simulink model "rl_with_free"  (R2021a)
settings: Solver=ode3  StartTime=0.0  StopTime=no_of_cycles/freq  MaxStep=1e-4  RelTol=1e-3
values from neighbouring files (symbols this model uses):
  firing_angle = c    [control.m]
  freq = a    [control.m]    (also in uncontrolled.m)
  peak_amp = d    [control.m]    (also in uncontrolled.m)
libraries: spsThyristorLib x4, spsACVoltageSourceLib x1, spsCurrentMeasurementLib x1, spsDiodeLib x1, spsSeriesRLCBranchLib x1, spsVoltageMeasurementLib x1, spspowerguiLib x1
settings Model: Creator=Souhardya  LastModifiedBy=sayan
settings SolverCC: AlgebraicLoopSolver=TrustRegion
settings DataIOCC: ReturnWorkspaceOutputs=off
settings DebuggingCC: SFMachineParentedDataDiag=warning  ArithmeticOperatorsInVariantConditions=warning
settings SFSimCC: SimUseLocalCustomCode=off  CustomCodeUndefinedFunction=UseInterfaceOnly
settings RTWCC: RTWUseLocalCustomCode=off
settings CodeAppCC: StateflowObjectComments=on
settings SimscapeCC: SimscapeNormalizeSystem=off

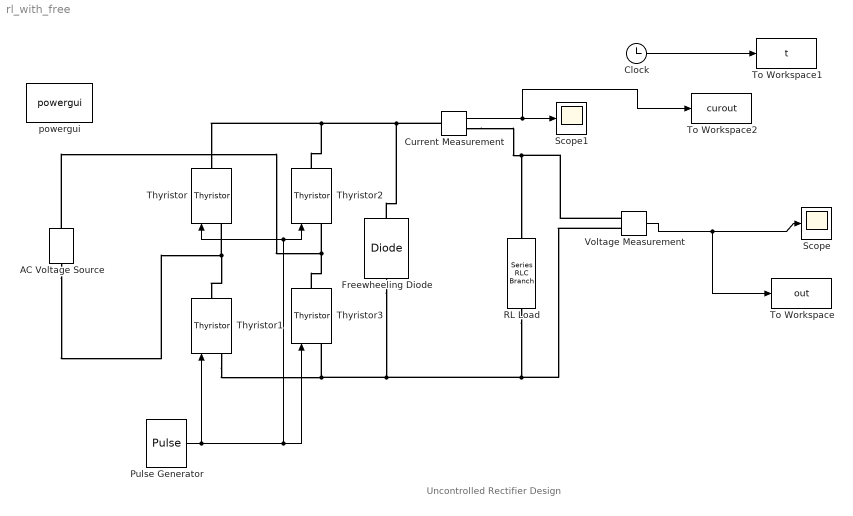
== system rl_with_free ==
  note: Uncontrolled Rectifier Design
  AC Voltage Source : spsACVoltageSourceLib/AC Voltage Source  Amplitude=peak_amp  Phase=0  Frequency=freq  SampleTime=0  Measurements=None  BusType=swing  Pref=10e3  Qref=0  Qmin=-inf  Qmax=+inf
  Clock : Clock
  Current Measurement : spsCurrentMeasurementLib/Current Measurement  PhasorSimulation=off  OutputType=Complex  PSBequivalent=0
  Freewheeling Diode : spsDiodeLib/Diode  Ron=0.001  Lon=0  Vf=0.8  IC=0  UseSnubber=0  Rs=500  Cs=250e-9  Measurements=off
  Pulse Generator : DiscretePulseGenerator  PulseType=Time based  Period=1/(2*freq)  PulseWidth=5  PhaseDelay=((1/freq)/360)*mod(firing_angle,360)
  RL Load : spsSeriesRLCBranchLib/Series RLC Branch  LConnTagsString=__new0  RConnTagsString=__new0  BranchType=RL  Resistance=1  Inductance=5e-2  SetiL0=off  InitialCurrent=0  Capacitance=1e-6  Setx0=off  InitialVoltage=0  Measurements=None
  Scope : Scope
  Scope1 : Scope
  Thyristor{,1..3} (4 alike) : spsThyristorLib/Thyristor  Ron=0.001  Lon=0  Vf=0.8  IC=0  Rs=500  Cs=250e-9  Measurements=off
  To Workspace : ToWorkspace  VariableName=out  SampleTime=-1
  To Workspace1 : ToWorkspace  VariableName=t  SampleTime=-1
  To Workspace2 : ToWorkspace  VariableName=curout  SampleTime=-1
  Voltage Measurement : spsVoltageMeasurementLib/Voltage Measurement  PhasorSimulation=off  OutputType=Complex  PSBequivalent=0
  powergui : spspowerguiLib/powergui  Priority=1  SimulationMode=Continuous  SampleTime=50e-6  frequency=60  Iterations=50  frequencyindice=0  Pbase=100e6  ErrMax=1e-4  UnitsV=kV  UnitsW=MW  buscounter=0  FunctionMessages=off  echomessages=off  EnableUseOfTLC=off  CurrentSourceSwitches=off  DisableSnubberDevices=off  DisableRonSwitches=off  DisableVfSwitches=off  DisplayEquations=off  AutomaticDiscreteSolvers=off  SolverType=Tustin/Backward Euler (TBE)  Interpol=off  ExternalGateDelay=off  methode=off  Ts=100  x0status=blocks  SPID=on  SwTol=0  HookPort=off  NonlinearTolerance=1e-4  nMaxIteration=100  ContinueOnMaxIteration=off  RestoreLinks=warning  ResistiveCurrentMeasurement=off  Frange=[0:2:500]  Ylog=off  Xlog=on  ShowGrid=off  save=off  variable=ZData  structure=0  ZoomFFT=off  StartTime=0.0  cycles=1  DisplayStyle=1  fundamental=60  FreqAxis=off  MaxFrequency=1000  frequencyindicesteady=1  RmsSteady=1  display=off
  wires:
  Clock/1 -> To Workspace1/1
  Pulse Generator/1 -> Thyristor2/1, Thyristor/1, Thyristor3/1, Thyristor1/1
  Voltage Measurement/1 -> To Workspace/1, Scope/1
  Current Measurement/1 -> To Workspace2/1, Scope1/1
  connections:
  Thyristor3/LConn1 -- Voltage Measurement/LConn2 -- RL Load/RConn1 -- Freewheeling Diode/LConn1 -- Thyristor1/LConn1
  Thyristor/LConn1 -- AC Voltage Source/LConn1 -- Thyristor1/RConn1
  Thyristor3/RConn1 -- AC Voltage Source/RConn1 -- Thyristor2/LConn1
  Current Measurement/RConn1 -- Voltage Measurement/LConn1 -- RL Load/LConn1
  Thyristor2/RConn1 -- Freewheeling Diode/RConn1 -- Current Measurement/LConn1 -- Thyristor/RConn1
